simulink model "lab1sm"  (R2021a)
settings: Solver=VariableStepAuto  StartTime=0.0  StopTime=30  MinStep=1e-9  RelTol=1e-3  AbsTol=1e-3  EnableMultiTasking=on
undefined symbols (not defined in the file): b1, b2, b3, F_1, F_2, time_F_1, time_F_2, x1_0, x2_0
libraries: fl_lib x17, nesl_utility x13, sdl_lib x3
settings Model: Creator=Alex  LastModifiedBy=Alex
settings SolverCC: AutoScaleAbsTol=off  AlgebraicLoopSolver=TrustRegion
settings DataIOCC: LimitDataPoints=on  MaxDataPoints=10000
settings OptimizationCC: LifeSpan=inf
settings DebuggingCC: AllowSymbolicDim=off  SFUnexpectedBacktrackingDiag=warning  SFNoUnconditionalDefaultTransitionDiag=warning  SFExecutionAtInitializationDiag=none  SFMachineParentedDataDiag=warning  ArithmeticOperatorsInVariantConditions=warning
settings SFSimCC: SimUseLocalCustomCode=off  CustomCodeUndefinedFunction=UseInterfaceOnly
settings RTWCC: RTWUseLocalCustomCode=off
settings CodeAppCC: StateflowObjectComments=on
settings GRTTargetCC: TargetLangStandard=C89/C90 (ANSI)
settings ConfigComp: CovMetricSettings=dw  CovSaveCumulativeToWorkspaceVar=on  CovSaveSingleToWorkspaceVar=on  CovExternalEMLEnable=off  CovSFcnEnable=off
settings SimscapeCC: SimscapeLogType=all  SimscapeLogSimulationStatistics=on  SimscapeLogDataHistory=10000

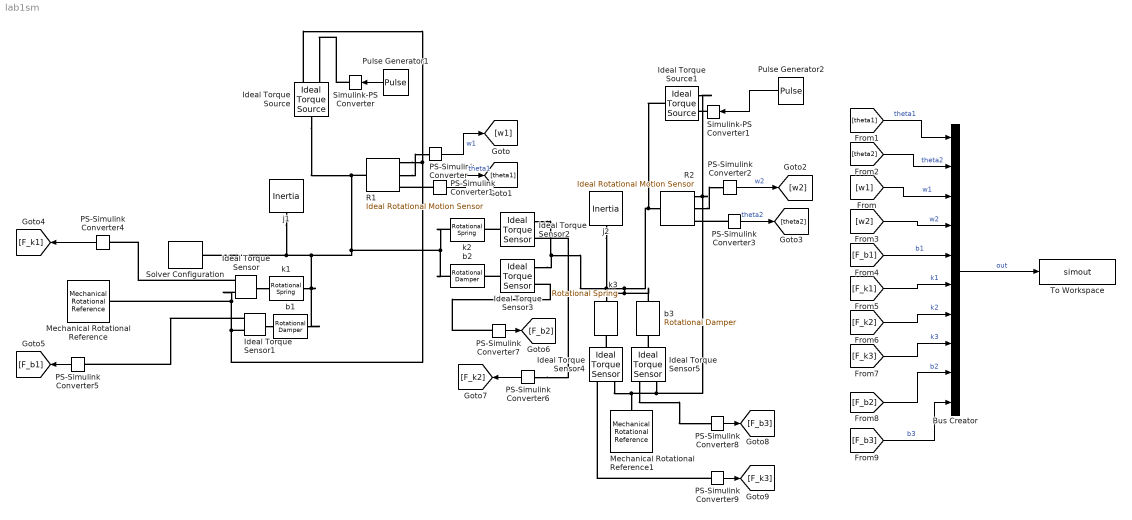
== system lab1sm ==
  Bus Creator : BusCreator  Inputs=10
  Ideal Torque Sensor{,1..5} (6 alike) : fl_lib/Mechanical/Mechanical Sensors/Ideal Torque Sensor
  Ideal Torque Source : fl_lib/Mechanical/Mechanical Sources/Ideal Torque Source
  Ideal Torque Source1 : fl_lib/Mechanical/Mechanical Sources/Ideal Torque Source
  Mechanical Rotational Reference : fl_lib/Mechanical/Rotational Elements/Mechanical Rotational Reference
  Mechanical Rotational Reference1 : fl_lib/Mechanical/Rotational Elements/Mechanical Rotational Reference
  PS-Simulink Converter{,1..9} (10 alike) : nesl_utility/PS-Simulink Converter  PhysicalDomain=network_engine_domain  SubClassName=ps_output  LeftPortType=input  RightPortType=output  PseudoPeriodic=off  Frequencies=[]  Unit=inherit  AffineConversion=off
      settings: SourceProductBaseCode=PW,SS
  Pulse Generator1 : DiscretePulseGenerator  PulseType=Time based  Amplitude=F_1  Period=t+10  PulseWidth=100 * time_F_1 / (t + 10)
  Pulse Generator2 : DiscretePulseGenerator  PulseType=Time based  Amplitude=F_2  Period=t+10  PulseWidth=100 * time_F_2 / (t + 10)
  R1 : fl_lib/Mechanical/Mechanical Sensors/Ideal Rotational Motion Sensor  wrap_angle=simscape.enum.onoff.off  offset=x1_0 rad
  R2 : fl_lib/Mechanical/Mechanical Sensors/Ideal Rotational Motion Sensor  wrap_angle=simscape.enum.onoff.off  offset=x2_0 rad
  Simulink-PS Converter : nesl_utility/Simulink-PS Converter  PhysicalDomain=network_engine_domain  SubClassName=ps_input  LeftPortType=input  RightPortType=output  PseudoPeriodic=off  Frequencies=[]  NoiseDistribution=none  NoiseParameters=[]  Unit=1  AffineConversion=off  FilteringAndDerivatives=provide  SimscapeFilterOrder=1  InputFilterTimeConstant=0.001  UdotUserProvided=0
      settings: SourceProductBaseCode=PW,SS
  Simulink-PS Converter1 : nesl_utility/Simulink-PS Converter  PhysicalDomain=network_engine_domain  SubClassName=ps_input  LeftPortType=input  RightPortType=output  PseudoPeriodic=off  Frequencies=[]  NoiseDistribution=none  NoiseParameters=[]  Unit=1  AffineConversion=off  FilteringAndDerivatives=provide  SimscapeFilterOrder=1  InputFilterTimeConstant=0.001  UdotUserProvided=0
      settings: SourceProductBaseCode=PW,SS
  Solver Configuration : nesl_utility/Solver Configuration  PhysicalDomain=network_engine_domain  SubClassName=solver  LeftPortType=input  RightPortType=generic  Tones=[]  Harmonics=[]  SimulateNoise=off  Profile=off  UseLocalSampling=off  EnableSwitchedLinearOptims=on  FrequencyDomain=off  UseCCode=off  RelTol=0.001  AbsTol=1e-06  MinStep=1e-09  ToWorkspace=off  RevertToSquareIcSolve=off  NumHomotopyIterations=100  PhasorMode=off  PhasorModeNumHarmonics=1  DoDC=off  ResidualTolerance=1e-09  UseLocalSolver=off  LocalSolverChoice=NE_BACKWARD_EULER_ADVANCER  LocalSolverSampleTime=0.001  DoFixedCost=off  MaxNonlinIter=3  MaxModeIter=2  ComputeImpulses=off  ImpulseIterations=2  LinearAlgebra=Sparse  EquationFormulation=NE_TIME_EF  DelaysMemoryBudget=1024  AutomaticFiltering=on  FilteringTimeConstant=0.001  PartitionStorageMethod=AS_NEEDED  PartitionMemoryBudget=1024  PartitionMethod=FAST
      settings: SourceProductBaseCode=PW,SS
  To Workspace : ToWorkspace  VariableName=simout  SaveFormat=Timeseries  SampleTime=-1
  b1 : sdl_lib/Couplings & Drives/Springs & Dampers/Rotational Damper  D=b1 N*m/(rad/s)  enable_faults=0  b_fault=100 N*m/(rad/s)  temporal_fault=0  fault_time=5 s  shock_fault=0  acceleration_limit=100 rad/s^2  shock_limit=1  report_fault=1
      settings: SourceProductBaseCode=LD
  b2 : sdl_lib/Couplings & Drives/Springs & Dampers/Rotational Damper  D=b2 N*m/(rad/s)  enable_faults=0  b_fault=100 N*m/(rad/s)  temporal_fault=0  fault_time=5 s  shock_fault=0  acceleration_limit=100 rad/s^2  shock_limit=1  report_fault=1
      settings: SourceProductBaseCode=LD
  b3 : sdl_lib/Couplings & Drives/Springs & Dampers/Rotational Damper  D=b3 N*m/(rad/s)  enable_faults=0  b_fault=100 N*m/(rad/s)  temporal_fault=0  fault_time=5 s  shock_fault=0  acceleration_limit=100 rad/s^2  shock_limit=1  report_fault=1
      settings: SourceProductBaseCode=LD
  j1 : fl_lib/Mechanical/Rotational Elements/Inertia  inertia=j1 kg*m^2  num_ports=foundation.enum.numPorts2.one  w_specify=off  w_priority=High  w=0 rad/s  w_nominal_specify=off  w_nominal_unit=rad/s  w_nominal_value=1  t_specify=off  t_priority=None  t=0 N*m  t_nominal_specify=off  t_nominal_unit=N*m  t_nominal_value=1
  j2 : fl_lib/Mechanical/Rotational Elements/Inertia  inertia=j2 kg*m^2  num_ports=foundation.enum.numPorts2.one  w_specify=off  w_priority=High  w=0 rad/s  w_nominal_specify=off  w_nominal_unit=rad/s  w_nominal_value=1  t_specify=off  t_priority=None  t=0 N*m  t_nominal_specify=off  t_nominal_unit=N*m  t_nominal_value=1
  k1 : fl_lib/Mechanical/Rotational Elements/Rotational Spring  spr_rate=k1 N*m/rad  w_specify=off  w_priority=None  w=0 rad/s  w_nominal_specify=off  w_nominal_unit=rad/s  w_nominal_value=1  t_specify=off  t_priority=None  t=0 N*m  t_nominal_specify=off  t_nominal_unit=N*m  t_nominal_value=1  phi_specify=on  phi_priority=High  phi=x1_0 rad  phi_nominal_specify=off  phi_nominal_unit=rad  phi_nominal_value=1
  k2 : fl_lib/Mechanical/Rotational Elements/Rotational Spring  spr_rate=k2 N*m/rad  w_specify=off  w_priority=None  w=0 rad/s  w_nominal_specify=off  w_nominal_unit=rad/s  w_nominal_value=1  t_specify=off  t_priority=None  t=0 N*m  t_nominal_specify=off  t_nominal_unit=N*m  t_nominal_value=1  phi_specify=on  phi_priority=High  phi=x2_0 - x1_0 rad  phi_nominal_specify=off  phi_nominal_unit=rad  phi_nominal_value=1
  k3 : fl_lib/Mechanical/Rotational Elements/Rotational Spring  spr_rate=k3 N*m/rad  w_specify=off  w_priority=None  w=0 rad/s  w_nominal_specify=off  w_nominal_unit=rad/s  w_nominal_value=1  t_specify=off  t_priority=None  t=0 N*m  t_nominal_specify=off  t_nominal_unit=N*m  t_nominal_value=1  phi_specify=on  phi_priority=High  phi=x2_0 rad  phi_nominal_specify=off  phi_nominal_unit=rad  phi_nominal_value=1
  wires:
  Bus Creator/1 -> To Workspace/1  "out"
  PS-Simulink Converter/1 -> [w1]  "w1"
  PS-Simulink Converter1/1 -> [theta1]  "theta1"
  [theta1] -> Bus Creator/1  "theta1"
  [w1] -> Bus Creator/3  "w1"
  [theta2] -> Bus Creator/2  "theta2"
  PS-Simulink Converter3/1 -> [theta2]  "theta2"
  PS-Simulink Converter2/1 -> [w2]  "w2"
  Pulse Generator1/1 -> Simulink-PS Converter/1
  Pulse Generator2/1 -> Simulink-PS Converter1/1
  PS-Simulink Converter4/1 -> [F_k1]
  PS-Simulink Converter5/1 -> [F_b1]
  [w2] -> Bus Creator/4  "w2"
  [F_b1] -> Bus Creator/5  "b1"
  [F_k1] -> Bus Creator/6  "k1"
  PS-Simulink Converter6/1 -> [F_k2]
  PS-Simulink Converter7/1 -> [F_b2]
  PS-Simulink Converter8/1 -> [F_b3]
  PS-Simulink Converter9/1 -> [F_k3]
  [F_k2] -> Bus Creator/7  "k2"
  [F_k3] -> Bus Creator/8  "k3"
  [F_b2] -> Bus Creator/9  "b2"
  [F_b3] -> Bus Creator/10  "b3"
  connections:
  R1/RConn1 -- Ideal Torque Sensor/RConn1 -- Mechanical Rotational Reference/LConn1 -- Ideal Torque Sensor1/RConn1 -- Ideal Torque Source/RConn2
  b2/RConn1 -- R1/LConn1 -- Ideal Torque Source/LConn1 -- b1/LConn1 -- k1/LConn1 -- Solver Configuration/RConn1 -- j1/LConn1 -- k2/RConn1
  R1/RConn2 -- PS-Simulink Converter/LConn1
  PS-Simulink Converter1/LConn1 -- R1/RConn3
  Ideal Torque Sensor3/RConn1 -- Ideal Torque Sensor2/RConn1 -- j2/LConn1 -- b3/LConn1 -- k3/LConn1 -- Ideal Torque Source1/LConn1 -- R2/LConn1
  R2/RConn2 -- PS-Simulink Converter2/LConn1
  PS-Simulink Converter3/LConn1 -- R2/RConn3
  R2/RConn1 -- Ideal Torque Sensor5/RConn1 -- Ideal Torque Sensor4/RConn1 -- Mechanical Rotational Reference1/LConn1 -- Ideal Torque Source1/RConn2
  Simulink-PS Converter/RConn1 -- Ideal Torque Source/RConn1
  Simulink-PS Converter1/RConn1 -- Ideal Torque Source1/RConn1
  Ideal Torque Sensor/LConn1 -- k1/RConn1
  Ideal Torque Sensor/RConn2 -- PS-Simulink Converter4/LConn1
  Ideal Torque Sensor1/LConn1 -- b1/RConn1
  Ideal Torque Sensor1/RConn2 -- PS-Simulink Converter5/LConn1
  Ideal Torque Sensor2/LConn1 -- k2/LConn1
  Ideal Torque Sensor3/LConn1 -- b2/LConn1
  PS-Simulink Converter7/LConn1 -- Ideal Torque Sensor3/RConn2
  Ideal Torque Sensor4/LConn1 -- k3/RConn1
  Ideal Torque Sensor5/LConn1 -- b3/RConn1
  Ideal Torque Sensor5/RConn2 -- PS-Simulink Converter8/LConn1
  PS-Simulink Converter9/LConn1 -- Ideal Torque Sensor4/RConn2
  PS-Simulink Converter6/LConn1 -- Ideal Torque Sensor2/RConn2
